simulink model "unicycle_simulation"  (R2013a)
settings: Solver=ode45  StartTime=0.0  StopTime=10.0  RelTol=1e-3
settings Model: Creator=Paresh  LastModifiedBy=Paresh

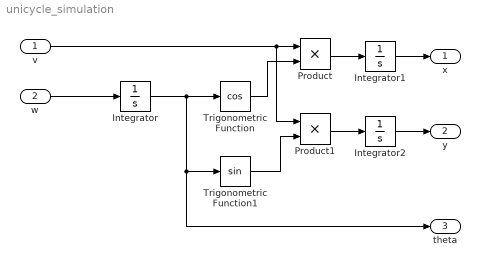
== system unicycle_simulation ==
  v : Inport
  w : Inport  Port=2
  Integrator : Integrator
  Integrator1 : Integrator
  Integrator2 : Integrator
  Product : Product
  Product1 : Product
  Trigonometric Function : Trigonometry  Operator=cos
  Trigonometric Function1 : Trigonometry
  x : Outport
  y : Outport  Port=2
  theta : Outport  Port=3
  wires:
  v/1 -> Product1/1, Product/1
  w/1 -> Integrator/1
  Integrator/1 -> theta/1, Trigonometric Function1/1, Trigonometric Function/1
  Trigonometric Function/1 -> Product/2
  Trigonometric Function1/1 -> Product1/2
  Product/1 -> Integrator1/1
  Integrator1/1 -> x/1
  Product1/1 -> Integrator2/1
  Integrator2/1 -> y/1
